simulink model "Drone_2D"  (R2020a)
settings: Solver=FixedStepAuto  StartTime=0.0  StopTime=100  FixedStep=0.01  RelTol=1e-3
values from neighbouring files (symbols this model uses):
  g = -9.81    [SetWorkspace.m]
  m = 0.2    [SetWorkspace.m]
  ts = 0.01    [SetWorkspace.m]    (also in signal.m = 0.1)
libraries: simulink x27
(part 2 of 2)

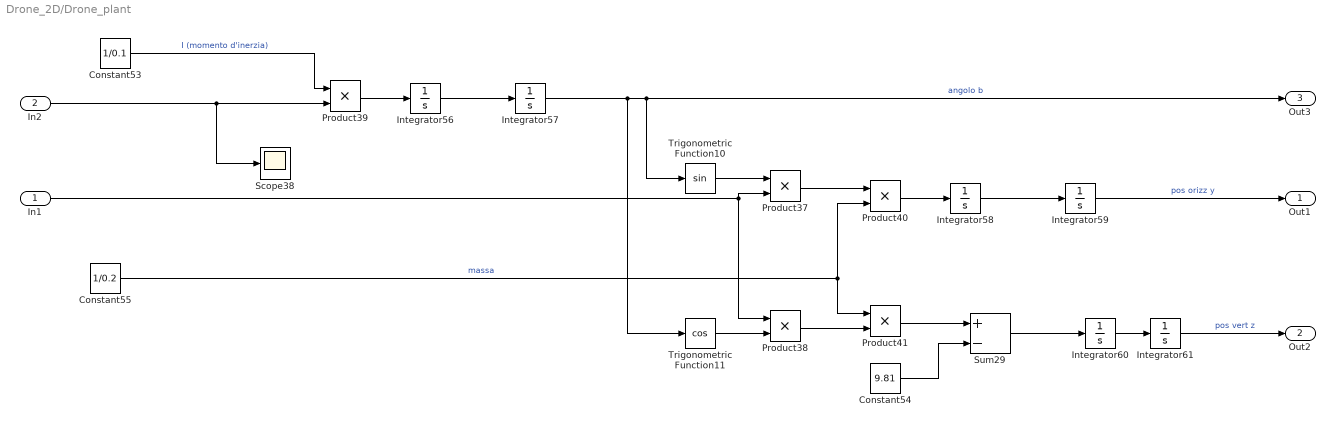
== system Drone_2D/Drone_plant ==
  In1 : Inport  Tag=torque  Description=torque
  In2 : Inport  Tag=thrust  Description=thrust  Port=2
  Constant53 : Constant  Value=1/0.1
  Constant54 : Constant  Value=9.81
  Constant55 : Constant  Value=1/0.2
  Integrator{56..61} (6 alike) : Integrator
  Product{37..41} (5 alike) : Product
  Scope38 : Scope
  Sum29 : Sum  Inputs=+-
  Trigonometric Function10 : Trigonometry
  Trigonometric Function11 : Trigonometry  Operator=cos
  Out1 : Outport  Tag=y position  Description=y position
  Out2 : Outport  Tag=z position  Description=z position  Port=2
  Out3 : Outport  Tag=roll angle  Description=roll angle  Port=3
  wires:
  Integrator60/1 -> Integrator61/1
  In1/1 -> Product38/1, Product37/2
  Sum29/1 -> Integrator60/1
  Integrator56/1 -> Integrator57/1
  Product39/1 -> Integrator56/1
  In2/1 -> Scope38/1, Product39/2
  Integrator57/1 -> Trigonometric Function11/1, Out3/1, Trigonometric Function10/1  "angolo b"
  Product38/1 -> Product41/2
  Constant55/1 -> Product40/2, Product41/1  "massa"
  Product40/1 -> Integrator58/1
  Integrator58/1 -> Integrator59/1
  Product41/1 -> Sum29/1
  Trigonometric Function11/1 -> Product38/2
  Constant54/1 -> Sum29/2
  Trigonometric Function10/1 -> Product37/1
  Product37/1 -> Product40/1
  Integrator61/1 -> Out2/1  "pos vert z"
  Constant53/1 -> Product39/1  "I (momento d'inerzia)"
  Integrator59/1 -> Out1/1  "pos orizz y"
